simulink subsystem "visualization_ctrl"  (R2026a)
settings: Solver=VariableStepAuto
undefined symbols (not defined in the file): act_gear_ratio
libraries: simulink_extras x2
settings Model: Creator=finnb  LastModifiedBy=trist

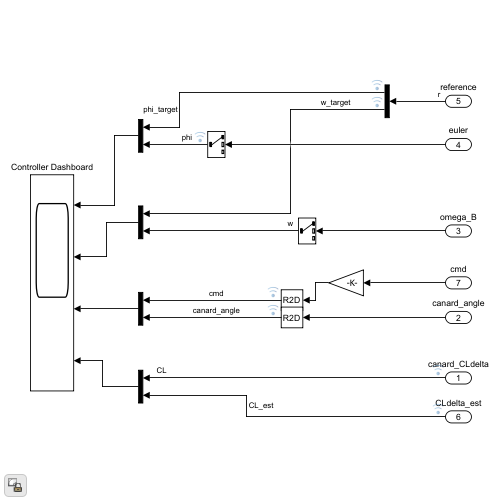
[thumbnail: Simulink's stored preview of the top-level diagram]
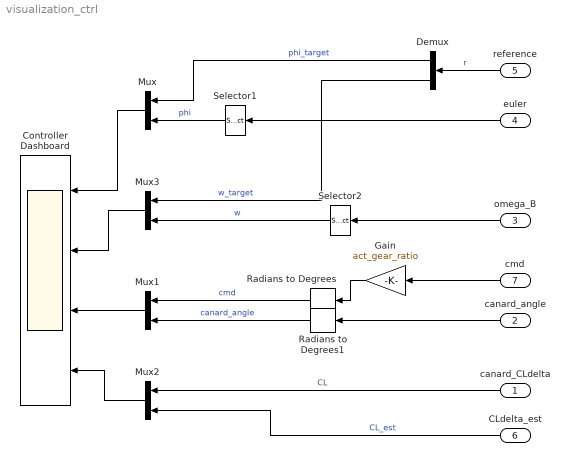
== system visualization_ctrl ==
  canard_CLdelta : Inport
  canard_angle : Inport  Port=2
  omega_B : Inport  Port=3
  euler : Inport  Port=4
  reference : Inport  Port=5  PortDimensions=2
  CLdelta_est : Inport  Port=6
  cmd : Inport  Port=7
  Controller Dashboard : Scope  NumInputPorts=4
      settings: ActiveDisplayString=4  Title=Roll Control Coefficient derivative%<SignalLabel>  ActiveDisplayYMinimum=-2.9040994808204914  ActiveDisplayYMaximum=3.3014318182316078  DataLoggingVariableName=ScopeData7
  Demux : Demux  Outputs=2
  Gain : Gain  Gain=act_gear_ratio
  Mux{,1..3} (4 alike) : Mux  Inputs=2
  Radians to Degrees : simulink_extras/Transformations/Radians to Degrees
  Radians to Degrees1 : simulink_extras/Transformations/Radians to Degrees
  Selector1 : Selector  InputPortWidth=3  IndexOptions=Index vector (dialog)  Indices=[1]  OutputSizes=1
  Selector2 : Selector  InputPortWidth=3  IndexOptions=Index vector (dialog)  Indices=[1]  OutputSizes=1
  wires:
  euler/1 -> Selector1/1
  Mux/1 -> Controller Dashboard/1
  Selector1/1 -> Mux/2  "phi"
  canard_angle/1 -> Radians to Degrees1/1
  Mux1/1 -> Controller Dashboard/3
  CLdelta_est/1 -> Mux2/2  "CL_est"
  canard_CLdelta/1 -> Mux2/1  "CL"
  Mux2/1 -> Controller Dashboard/4
  Radians to Degrees/1 -> Mux1/1  "cmd"
  Radians to Degrees1/1 -> Mux1/2  "canard_angle"
  cmd/1 -> Gain/1
  Gain/1 -> Radians to Degrees/1
  omega_B/1 -> Selector2/1
  Demux/1 -> Mux/1  "phi_target"
  Selector2/1 -> Mux3/2  "w"
  Demux/2 -> Mux3/1  "w_target"
  Mux3/1 -> Controller Dashboard/2
  reference/1 -> Demux/1  "r"
